simulink model "OfflineTestbench_OpenLoop"  (R2019b)
settings: Solver=ode1  StartTime=0.0  StopTime=30  FixedStep=0.01  RelTol=1e-3
PostLoadFcn:
  | , if any(exist('dsrtsu_mdlpostloadfcn', 'file') == [2, 3, 6]), try dsrtsu_mdlpostloadfcn('Execute', bdroot); catch fprintf('Error in PostLoadFcn (dsrtsu_mdlpostloadfcn) for model "%s":\n %s\n', bdroot, lasterr); end, end,
undefined symbols (not defined in the file): default_localization_bus, default_vehicle_state_bus, localization_testbed_matrix, MeasurementTime, Motion, Pose, Steering, time_testbed_vector, trajectory_testbed_matrix, vehicle_can_testbed_matrix
libraries: Lib_VehicleModel x3, Lib_Controller x1
settings Model: DSRTSU_INTERNAL_RTI_VER=550  DSRTSU_INTERNAL_RTI_TYPE=rti1401  RTICANMMDATA=struct('GeneralSetupData',struct('modelroot','C:\Users\kessler\Documents\fav\apollo_opensource\modules\autobox_control\models','generalsettings',struct('filesettings',struct('destfolder',struct('Name','RTICANMM_FILES','Check',1),'buildfolder',struct('Name','.','Check',1),'AbsDestfolder',struct('Name','C:\Users\kessler\Documents\fav\apollo_opensource\modules\autobox_control\models\RTICANMM_FILES'),'AbsBuildfolder',struct('Name','C:\Users\kessler\Documents\fav\apollo_opensource\modules\autobox_control\models'))),'options',struct('addpaths',1,'rmpaths',1,'addtrcexclusion',true,'cannavigator',struct('checkmonitoring',0),'show_usrtrc',0,'use_usrtrc',0),'advanced',struct('options',ones(1,100)),'MPSetup',{{}},'RTI',struct('Type','GRT','Ver','','Date',''),'modelname','OfflineTestbench_OpenLoop','block','OfflineTestbench_OpenLoop'))  DSRTSU_INTERNAL_RTIFPGA=150  Creator=esterle  LastModifiedBy=kessler
settings DataIOCC: ReturnWorkspaceOutputs=off
settings DebuggingCC: ArithmeticOperatorsInVariantConditions=warning
settings SFSimCC: SimUseLocalCustomCode=off  CustomCodeUndefinedFunction=UseInterfaceOnly
settings RTWCC: RTWUseLocalCustomCode=off

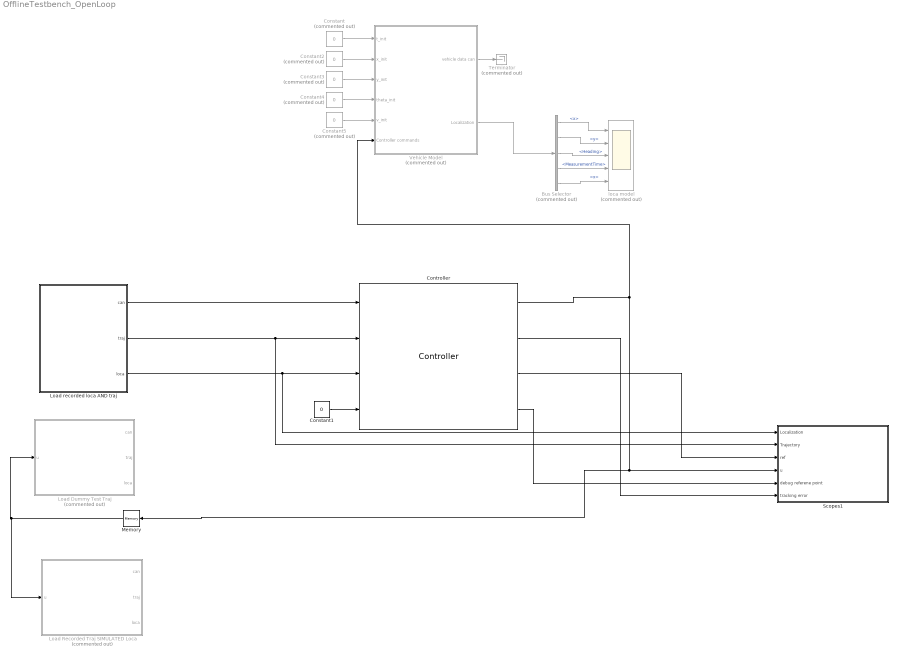
== system OfflineTestbench_OpenLoop ==
  Bus Selector : BusSelector  Commented=on  OutputSignals=Pose.Position.x,Pose.Position.y,Pose.Heading,MeasurementTime,Pose.LinearVelocity.x
  Constant{,2..5} (5 alike) : Constant  Commented=on  Value=0
  Constant1 : Constant  Value=0  OutDataTypeStr=boolean
  Controller : Lib_Controller/Controller  SystemSampleTime=-1  Latency=0  AutoFrameSizeCalculation=off
  Load Dummy Test Traj : Subsystem  Commented=on
  Load Recorded Traj SIMULATED Loca : Subsystem  Commented=on
  Load recorded loca AND traj : Subsystem
  Memory : Memory
  Scopes1 : Subsystem
  Terminator : Terminator  Commented=on
  Vehicle Model : Subsystem  Commented=on
  loca model : Scope  Commented=on  NumInputPorts=5
  wires:
  Constant1/1 -> Controller/4
  Controller/2 -> Scopes1/6(tracking error)
  Controller/1 -> Memory/1, Scopes1/4(u), Vehicle Model/6(Controller commands)
  Memory/1 -> Load Recorded Traj SIMULATED Loca/1(u), Load Dummy Test Traj/1(u)
  Controller/4 -> Scopes1/5(debug referene point)
  Controller/3 -> Scopes1/3(ref)
  Constant/1 -> Vehicle Model/1(t_init)
  Constant2/1 -> Vehicle Model/2(x_init)
  Constant3/1 -> Vehicle Model/3(y_init)
  Constant4/1 -> Vehicle Model/4(theta_init)
  Constant5/1 -> Vehicle Model/5(v_init)
  Vehicle Model/2(Localization) -> Bus Selector/1
  Vehicle Model/1(vehicle data can) -> Terminator/1
  Bus Selector/4 -> loca model/4  "<MeasurementTime>"
  Bus Selector/3 -> loca model/3  "<Heading>"
  Bus Selector/5 -> loca model/5  "<x>"
  Bus Selector/2 -> loca model/2  "<y>"
  Bus Selector/1 -> loca model/1  "<x>"
  Load recorded loca AND traj/2(traj) -> Scopes1/2(Trajectory), Controller/2
  Load recorded loca AND traj/3(loca) -> Scopes1/1(Localization), Controller/3
  Load recorded loca AND traj/1(can) -> Controller/1

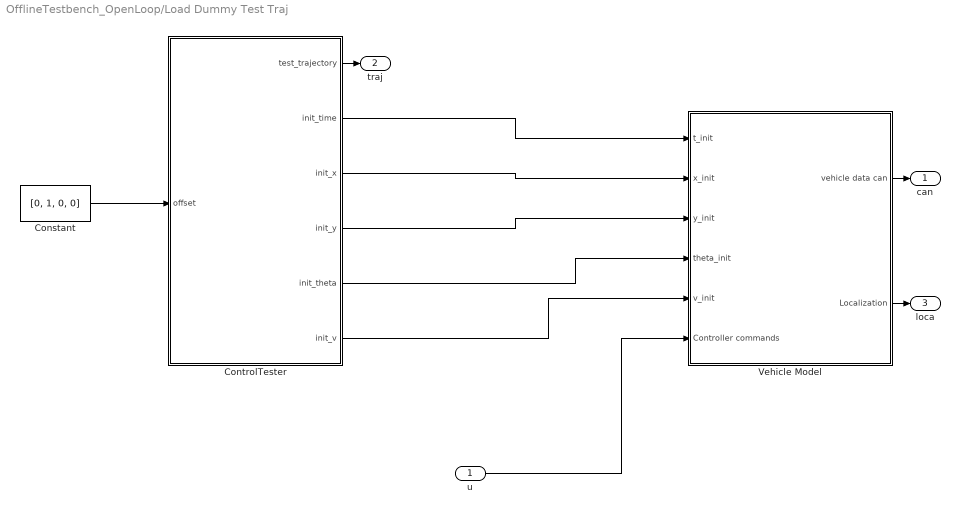
== system OfflineTestbench_OpenLoop/Load Dummy Test Traj ==
  u : Inport
  Constant : Constant  Value=[0, 1, 0, 0]
  "ControlTester " : MATLAB Function  TreatAsAtomicUnit=on
  Vehicle Model : Subsystem
  can : Outport  VectorParamsAs1DForOutWhenUnconnected=off
  traj : Outport  Port=2  VectorParamsAs1DForOutWhenUnconnected=off
  loca : Outport  Port=3  VectorParamsAs1DForOutWhenUnconnected=off
  wires:
  "ControlTester "/2(init_time) -> Vehicle Model/1(t_init)
  "ControlTester "/5(init_theta) -> Vehicle Model/4(theta_init)
  Constant/1 -> "ControlTester "/1(offset)
  "ControlTester "/6(init_v) -> Vehicle Model/5(v_init)
  "ControlTester "/3(init_x) -> Vehicle Model/2(x_init)
  "ControlTester "/4(init_y) -> Vehicle Model/3(y_init)
  "ControlTester "/1(test_trajectory) -> traj/1
  Vehicle Model/1(vehicle data can) -> can/1
  Vehicle Model/2(Localization) -> loca/1
  u/1 -> Vehicle Model/6(Controller commands)

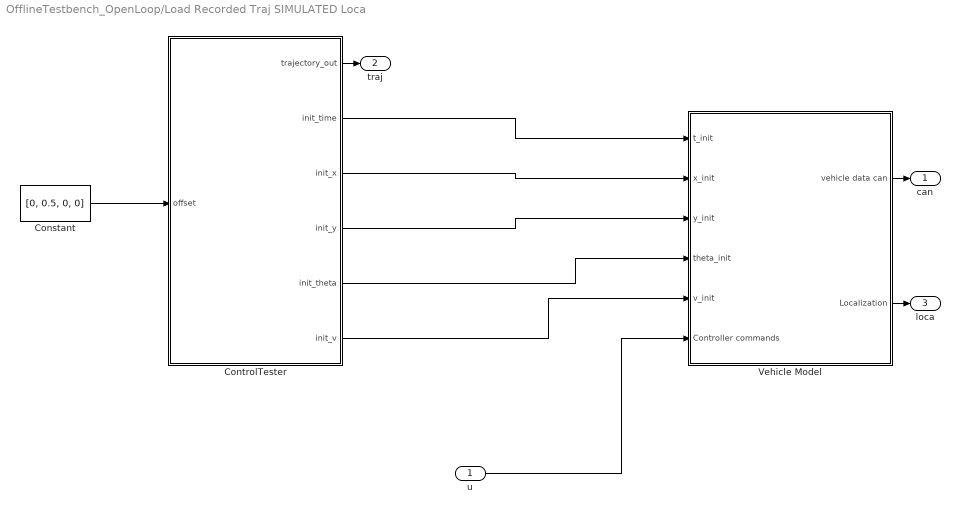
== system OfflineTestbench_OpenLoop/Load Recorded Traj SIMULATED Loca ==
  u : Inport
  Constant : Constant  Value=[0, 0.5, 0, 0]
  "ControlTester " : MATLAB Function  TreatAsAtomicUnit=on
  Vehicle Model : Subsystem
  can : Outport  VectorParamsAs1DForOutWhenUnconnected=off
  traj : Outport  Port=2  VectorParamsAs1DForOutWhenUnconnected=off
  loca : Outport  Port=3  VectorParamsAs1DForOutWhenUnconnected=off
  wires:
  u/1 -> Vehicle Model/6(Controller commands)
  Vehicle Model/2(Localization) -> loca/1
  Vehicle Model/1(vehicle data can) -> can/1
  "ControlTester "/1(trajectory_out) -> traj/1
  "ControlTester "/4(init_y) -> Vehicle Model/3(y_init)
  "ControlTester "/3(init_x) -> Vehicle Model/2(x_init)
  "ControlTester "/6(init_v) -> Vehicle Model/5(v_init)
  Constant/1 -> "ControlTester "/1(offset)
  "ControlTester "/5(init_theta) -> Vehicle Model/4(theta_init)
  "ControlTester "/2(init_time) -> Vehicle Model/1(t_init)

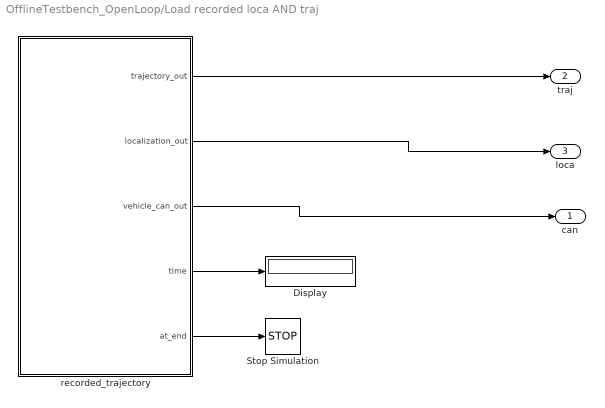
== system OfflineTestbench_OpenLoop/Load recorded loca AND traj ==
  Display : Display
  Stop Simulation : Stop
  recorded_trajectory : MATLAB Function  TreatAsAtomicUnit=on
  can : Outport  VectorParamsAs1DForOutWhenUnconnected=off
  traj : Outport  Port=2  VectorParamsAs1DForOutWhenUnconnected=off
  loca : Outport  Port=3  VectorParamsAs1DForOutWhenUnconnected=off
  wires:
  recorded_trajectory/5(at_end) -> Stop Simulation/1
  recorded_trajectory/4(time) -> Display/1
  recorded_trajectory/3(vehicle_can_out) -> can/1
  recorded_trajectory/2(localization_out) -> loca/1
  recorded_trajectory/1(trajectory_out) -> traj/1

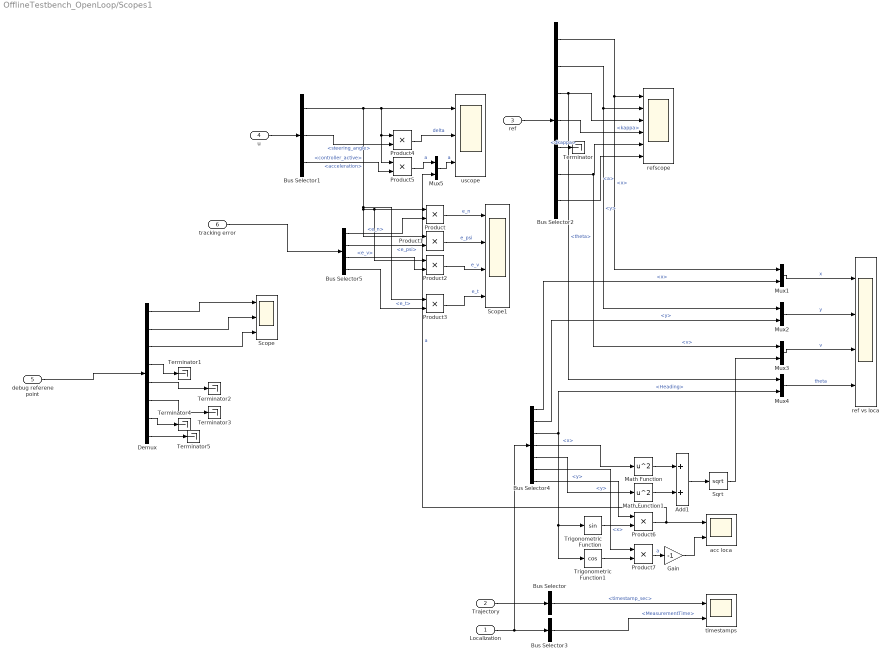
== system OfflineTestbench_OpenLoop/Scopes1 ==
  Localization : Inport  OutDataTypeStr=Bus: LocalizationToAutobox  BusOutputAsStruct=on
  Trajectory : Inport  Port=2  OutDataTypeStr=Bus: ControlTrajectory  BusOutputAsStruct=on
  ref : Inport  Port=3
  u : Inport  Port=4
  debug referene point : Inport  Port=5
  tracking error : Inport  Port=6
  Add1 : Sum
  Bus Selector : BusSelector  OutputSignals=timestamp_sec
  Bus Selector1 : BusSelector  OutputSignals=controller_active,steering_angle,acceleration
  Bus Selector2 : BusSelector  OutputSignals=x,y,theta,kappa,dkappa,v,a
  Bus Selector3 : BusSelector  OutputSignals=MeasurementTime
  Bus Selector4 : BusSelector  OutputSignals=Pose.Position.x,Pose.Position.y,Pose.Heading,Pose.LinearVelocity.x,Pose.LinearVelocity.y,Pose.LinearAcceleration.x,Pose.LinearAcceleration.y
  Bus Selector5 : BusSelector  OutputSignals=e_n,e_psi,e_v,e_t
  Demux : Demux  Outputs=8
  Gain : Gain  Gain=-1
  Math Function : Math  Operator=square  SaturateOnIntegerOverflow=on
  Math Function1 : Math  Operator=square  SaturateOnIntegerOverflow=on
  Mux{1..5} (5 alike) : Mux  Inputs=2
  Product{,1..7} (8 alike) : Product
  Scope : Scope  NumInputPorts=3
  Scope1 : Scope  NumInputPorts=4
  Sqrt : Sqrt  SaturateOnIntegerOverflow=on
  Terminator{,1..5} (6 alike) : Terminator
  Trigonometric Function : Trigonometry
  Trigonometric Function1 : Trigonometry  Operator=cos
  acc loca : Scope  NumInputPorts=2
  ref vs loca : Scope  NumInputPorts=4
  refscope : Scope  NumInputPorts=6
  timestamps : Scope  NumInputPorts=2
  uscope : Scope  NumInputPorts=3
  wires:
  Bus Selector1/1 -> Product3/1, Product2/1, Product/1, Product1/1, Product5/1, Product4/1, uscope/1  "<controller_active>"
  Bus Selector1/2 -> Product4/2  "<steering_angle>"
  Bus Selector1/3 -> Product5/2  "<acceleration>"
  Bus Selector2/5 -> Terminator/1  "<dkappa>"
  u/1 -> Bus Selector1/1
  ref/1 -> Bus Selector2/1
  Bus Selector2/4 -> refscope/4  "<kappa>"
  Bus Selector2/3 -> Mux4/1, refscope/3  "<theta>"
  Bus Selector2/1 -> Mux1/1, refscope/1  "<x>"
  Bus Selector2/6 -> Mux3/1, refscope/5  "<v>"
  Bus Selector2/7 -> refscope/6  "<a>"
  Bus Selector2/2 -> Mux2/1, refscope/2  "<y>"
  Trajectory/1 -> Bus Selector/1
  Localization/1 -> Bus Selector4/1, Bus Selector3/1
  Bus Selector3/1 -> timestamps/2  "<MeasurementTime>"
  Bus Selector/1 -> timestamps/1  "<timestamp_sec>"
  Mux4/1 -> ref vs loca/4  "theta"
  Mux2/1 -> ref vs loca/2  "y"
  Mux3/1 -> ref vs loca/3  "v"
  Mux1/1 -> ref vs loca/1  "x"
  Bus Selector4/1 -> Mux1/2  "<x>"
  Bus Selector4/2 -> Mux2/2  "<y>"
  Bus Selector4/3 -> Mux4/2, Trigonometric Function1/1, Trigonometric Function/1  "<Heading>"
  Math Function1/1 -> Add1/2
  Math Function/1 -> Add1/1
  Add1/1 -> Sqrt/1
  Bus Selector4/4 -> Math Function/1  "<x>"
  Bus Selector4/5 -> Math Function1/1  "<y>"
  Sqrt/1 -> Mux3/2
  Demux/3 -> Scope/3
  Demux/1 -> Scope/1
  Demux/2 -> Scope/2
  debug referene point/1 -> Demux/1
  Bus Selector5/2 -> Product1/2  "<e_psi>"
  Bus Selector5/4 -> Product3/2  "<e_t>"
  Bus Selector5/3 -> Product2/2  "<e_v>"
  Bus Selector5/1 -> Product/2  "<e_n>"
  tracking error/1 -> Bus Selector5/1
  Demux/4 -> Terminator1/1
  Demux/5 -> Terminator2/1
  Demux/6 -> Terminator3/1
  Demux/7 -> Terminator4/1
  Demux/8 -> Terminator5/1
  Product/1 -> Scope1/1  "e_n"
  Product1/1 -> Scope1/2  "e_psi"
  Product2/1 -> Scope1/3  "e_v"
  Product3/1 -> Scope1/4  "e_t"
  Product4/1 -> uscope/2  "delta"
  Product5/1 -> Mux5/1  "a"
  Mux5/1 -> uscope/3  "a"
  Trigonometric Function/1 -> Product6/2
  Bus Selector4/7 -> Product6/1  "<y>"
  Bus Selector4/6 -> Product7/1  "<x>"
  Trigonometric Function1/1 -> Product7/2
  Product6/1 -> Mux5/2, acc loca/1  "a"
  Product7/1 -> Gain/1  "a"
  Gain/1 -> acc loca/2

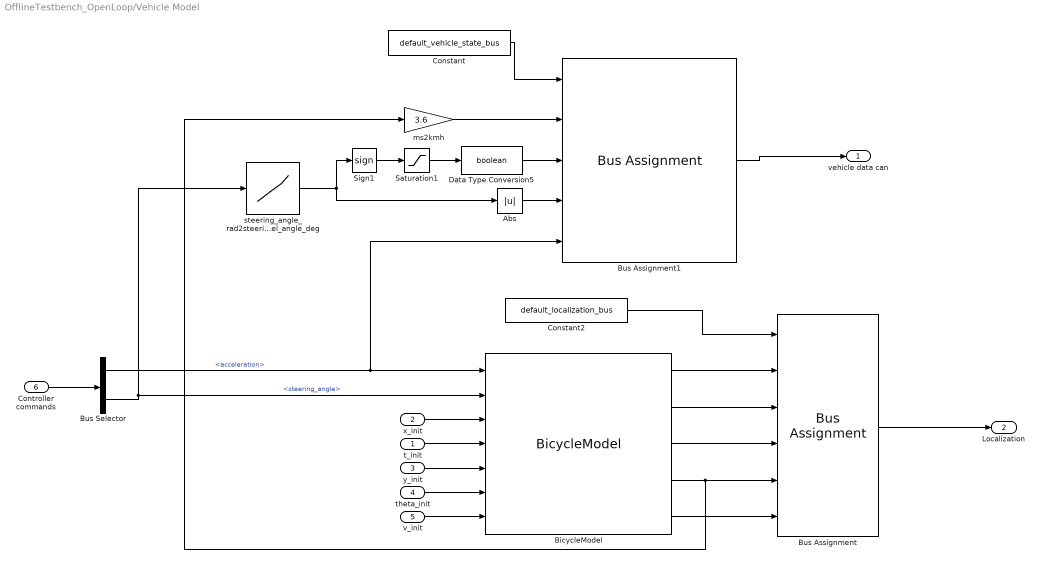
== system OfflineTestbench_OpenLoop/Vehicle Model ==
  t_init : Inport
  x_init : Inport  Port=2
  y_init : Inport  Port=3
  theta_init : Inport  Port=4
  v_init : Inport  Port=5
  Controller commands : Inport  Port=6
  Abs : Abs
  BicycleModel : Lib_VehicleModel/BicycleModel  l=2.6
  Bus Assignment : BusAssignment  AssignedSignals=Pose.Position.x,Pose.Position.y,Pose.Heading,Pose.LinearVelocity.x,MeasurementTime
  Bus Assignment1 : BusAssignment  AssignedSignals=Motion.VehicleVelocity,Steering.SteeringWheelAngleSign,Steering.SteeringWheelAngle,Motion.LongitudinalAcceleration
  Bus Selector : BusSelector  OutputSignals=acceleration,steering_angle
  Constant : Constant  Value=default_vehicle_state_bus  OutDataTypeStr=Bus: vehicle_data_can_bus
  Constant2 : Constant  Value=default_localization_bus  OutDataTypeStr=Bus: LocalizationToAutobox
  Data Type Conversion5 : DataTypeConversion  OutDataTypeStr=boolean
  Saturation1 : Saturate  UpperLimit=1  LowerLimit=0
  Sign1 : Signum
  ms2kmh : Gain  Gain=3.6
  steering_angle_rad2steering_wheel_angle_deg : Lookup_n-D  NumberOfTableDimensions=1  BreakpointsForDimension1=[-0.62 0 0.62]  Table=[-400, 0, 400]  InternalRulePriority=Speed  RndMeth=Simplest  InputSameDT=on
  vehicle data can : Outport  VectorParamsAs1DForOutWhenUnconnected=off
  Localization : Outport  Port=2  VectorParamsAs1DForOutWhenUnconnected=off
  wires:
  Controller commands/1 -> Bus Selector/1
  Bus Assignment/1 -> Localization/1
  Bus Selector/1 -> Bus Assignment1/5, BicycleModel/1  "<acceleration>"
  Bus Selector/2 -> BicycleModel/2, steering_angle_rad2steering_wheel_angle_deg/1  "<steering_angle>"
  BicycleModel/5 -> Bus Assignment/6
  y_init/1 -> BicycleModel/5
  BicycleModel/2 -> Bus Assignment/3
  BicycleModel/1 -> Bus Assignment/2
  BicycleModel/3 -> Bus Assignment/4
  v_init/1 -> BicycleModel/7
  theta_init/1 -> BicycleModel/6
  x_init/1 -> BicycleModel/3
  Constant2/1 -> Bus Assignment/1
  BicycleModel/4 -> Bus Assignment/5, ms2kmh/1
  t_init/1 -> BicycleModel/4
  Data Type Conversion5/1 -> Bus Assignment1/3
  Abs/1 -> Bus Assignment1/4
  Saturation1/1 -> Data Type Conversion5/1
  Sign1/1 -> Saturation1/1
  ms2kmh/1 -> Bus Assignment1/2
  steering_angle_rad2steering_wheel_angle_deg/1 -> Abs/1, Sign1/1
  Constant/1 -> Bus Assignment1/1
  Bus Assignment1/1 -> vehicle data can/1

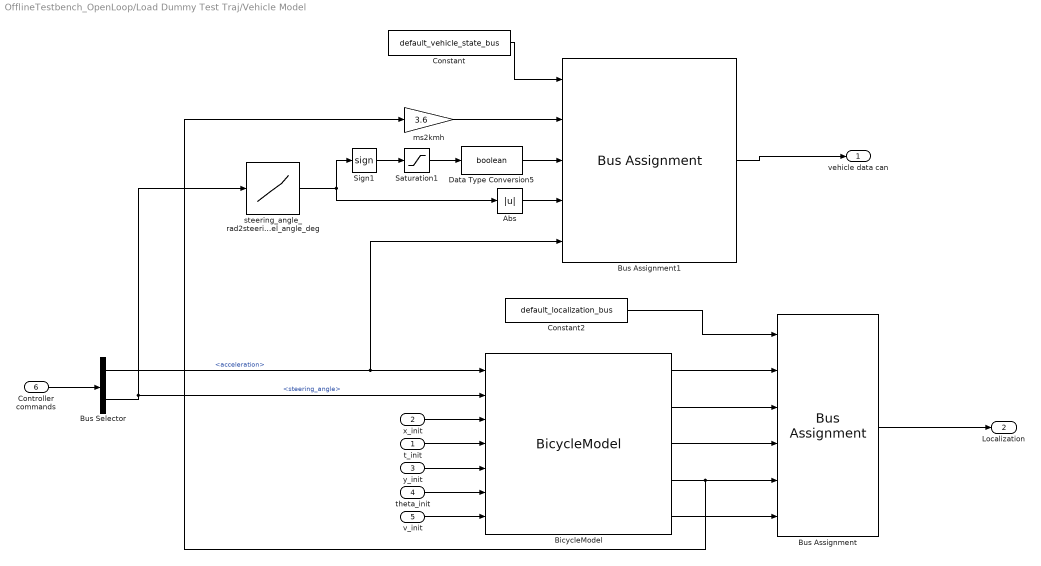
== system OfflineTestbench_OpenLoop/Load Dummy Test Traj/Vehicle Model ==
  t_init : Inport
  x_init : Inport  Port=2
  y_init : Inport  Port=3
  theta_init : Inport  Port=4
  v_init : Inport  Port=5
  Controller commands : Inport  Port=6
  Abs : Abs
  BicycleModel : Lib_VehicleModel/BicycleModel  l=2.6
  Bus Assignment : BusAssignment  AssignedSignals=Pose.Position.x,Pose.Position.y,Pose.Heading,Pose.LinearVelocity.x,MeasurementTime
  Bus Assignment1 : BusAssignment  AssignedSignals=Motion.VehicleVelocity,Steering.SteeringWheelAngleSign,Steering.SteeringWheelAngle,Motion.LongitudinalAcceleration
  Bus Selector : BusSelector  OutputSignals=acceleration,steering_angle
  Constant : Constant  Value=default_vehicle_state_bus  OutDataTypeStr=Bus: vehicle_data_can_bus
  Constant2 : Constant  Value=default_localization_bus  OutDataTypeStr=Bus: LocalizationToAutobox
  Data Type Conversion5 : DataTypeConversion  OutDataTypeStr=boolean
  Saturation1 : Saturate  UpperLimit=1  LowerLimit=0
  Sign1 : Signum
  ms2kmh : Gain  Gain=3.6
  steering_angle_rad2steering_wheel_angle_deg : Lookup_n-D  NumberOfTableDimensions=1  BreakpointsForDimension1=[-0.62 0 0.62]  Table=[-400, 0, 400]  InternalRulePriority=Speed  RndMeth=Simplest  InputSameDT=on
  vehicle data can : Outport  VectorParamsAs1DForOutWhenUnconnected=off
  Localization : Outport  Port=2  VectorParamsAs1DForOutWhenUnconnected=off
  wires:
  Controller commands/1 -> Bus Selector/1
  Bus Assignment/1 -> Localization/1
  Bus Selector/1 -> Bus Assignment1/5, BicycleModel/1  "<acceleration>"
  Bus Selector/2 -> BicycleModel/2, steering_angle_rad2steering_wheel_angle_deg/1  "<steering_angle>"
  BicycleModel/5 -> Bus Assignment/6
  y_init/1 -> BicycleModel/5
  BicycleModel/2 -> Bus Assignment/3
  BicycleModel/1 -> Bus Assignment/2
  BicycleModel/3 -> Bus Assignment/4
  v_init/1 -> BicycleModel/7
  theta_init/1 -> BicycleModel/6
  x_init/1 -> BicycleModel/3
  Constant2/1 -> Bus Assignment/1
  BicycleModel/4 -> Bus Assignment/5, ms2kmh/1
  t_init/1 -> BicycleModel/4
  Data Type Conversion5/1 -> Bus Assignment1/3
  Abs/1 -> Bus Assignment1/4
  Saturation1/1 -> Data Type Conversion5/1
  Sign1/1 -> Saturation1/1
  ms2kmh/1 -> Bus Assignment1/2
  steering_angle_rad2steering_wheel_angle_deg/1 -> Abs/1, Sign1/1
  Constant/1 -> Bus Assignment1/1
  Bus Assignment1/1 -> vehicle data can/1

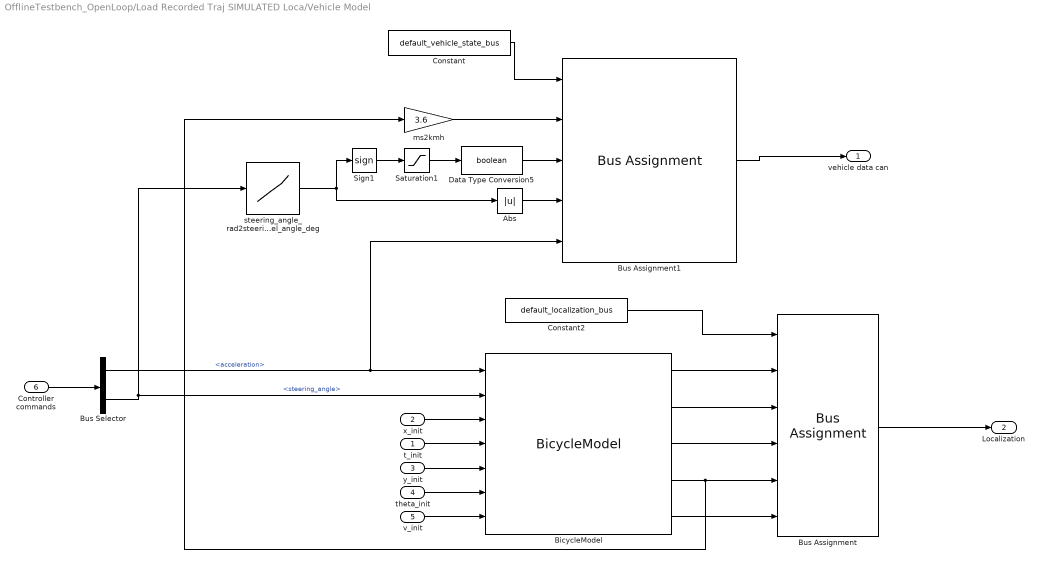
== system OfflineTestbench_OpenLoop/Load Recorded Traj SIMULATED Loca/Vehicle Model ==
  t_init : Inport
  x_init : Inport  Port=2
  y_init : Inport  Port=3
  theta_init : Inport  Port=4
  v_init : Inport  Port=5
  Controller commands : Inport  Port=6
  Abs : Abs
  BicycleModel : Lib_VehicleModel/BicycleModel  l=2.6
  Bus Assignment : BusAssignment  AssignedSignals=Pose.Position.x,Pose.Position.y,Pose.Heading,Pose.LinearVelocity.x,MeasurementTime
  Bus Assignment1 : BusAssignment  AssignedSignals=Motion.VehicleVelocity,Steering.SteeringWheelAngleSign,Steering.SteeringWheelAngle,Motion.LongitudinalAcceleration
  Bus Selector : BusSelector  OutputSignals=acceleration,steering_angle
  Constant : Constant  Value=default_vehicle_state_bus  OutDataTypeStr=Bus: vehicle_data_can_bus
  Constant2 : Constant  Value=default_localization_bus  OutDataTypeStr=Bus: LocalizationToAutobox
  Data Type Conversion5 : DataTypeConversion  OutDataTypeStr=boolean
  Saturation1 : Saturate  UpperLimit=1  LowerLimit=0
  Sign1 : Signum
  ms2kmh : Gain  Gain=3.6
  steering_angle_rad2steering_wheel_angle_deg : Lookup_n-D  NumberOfTableDimensions=1  BreakpointsForDimension1=[-0.62 0 0.62]  Table=[-400, 0, 400]  InternalRulePriority=Speed  RndMeth=Simplest  InputSameDT=on
  vehicle data can : Outport  VectorParamsAs1DForOutWhenUnconnected=off
  Localization : Outport  Port=2  VectorParamsAs1DForOutWhenUnconnected=off
  wires:
  Bus Assignment1/1 -> vehicle data can/1
  Constant/1 -> Bus Assignment1/1
  steering_angle_rad2steering_wheel_angle_deg/1 -> Sign1/1, Abs/1
  ms2kmh/1 -> Bus Assignment1/2
  Sign1/1 -> Saturation1/1
  Saturation1/1 -> Data Type Conversion5/1
  Abs/1 -> Bus Assignment1/4
  Data Type Conversion5/1 -> Bus Assignment1/3
  t_init/1 -> BicycleModel/4
  BicycleModel/4 -> ms2kmh/1, Bus Assignment/5
  Constant2/1 -> Bus Assignment/1
  x_init/1 -> BicycleModel/3
  theta_init/1 -> BicycleModel/6
  v_init/1 -> BicycleModel/7
  BicycleModel/3 -> Bus Assignment/4
  BicycleModel/1 -> Bus Assignment/2
  BicycleModel/2 -> Bus Assignment/3
  y_init/1 -> BicycleModel/5
  BicycleModel/5 -> Bus Assignment/6
  Bus Selector/2 -> steering_angle_rad2steering_wheel_angle_deg/1, BicycleModel/2  "<steering_angle>"
  Bus Selector/1 -> BicycleModel/1, Bus Assignment1/5  "<acceleration>"
  Bus Assignment/1 -> Localization/1
  Controller commands/1 -> Bus Selector/1

== matlab function OfflineTestbench_OpenLoop/Load Dummy Test Traj/ControlTester  ==
  data: test_trajectory output Bus: ControlTrajectory; init_time output; init_x output; init_y output; init_theta output; init_v output; offset input
function [test_trajectory, init_time, init_x, init_y, init_theta, init_v]  = ControlTester(offset)
coder.extrinsic('display')
persistent test_number;

test_trajectory = struct('n_trajectory_point',uint32(0),'x',zeros(1000,1), 'y',zeros(1000,1), ...
    'z', zeros(1000,1), 'theta', zeros(1000,1),'kappa',zeros(1000,1),...
    'dkappa', zeros(1000,1),'ddkappa', zeros(1000,1),'s',zeros(1000,1),...
    'v',zeros(1000,1),'a', zeros(1000,1),'relative_time',zeros(1000,1),...
    'timestamp_sec', zeros(1,1));

point3d = struct('x',double(0),'y',double(0),'z',double(0));
point_enu= struct('x',double(0),'y',double(0),'z',double(0));
quaternion = struct('qx',double(0),'qy',double(0),'qz',double(0),'qw',double(0));
pose = struct('Position',point_enu,'Orientation',quaternion,...
    'LinearVelocity',point3d,'LinearAcceleration',point3d, 'AngularVelocity',point3d,'Heading',double(0),...
    'LinearAccelerationVrf',point3d,'AngularVelocityVrf',point3d,'EulerAngles',point3d);
uncertainty = struct('PositionStdDev',point3d,'OrientationStdDev',point3d,...
'LinearVelocityStdDev',point3d,'LinearAccelerationStdDev',point3d,'AngularVelocityStdDev',point3d);

if isempty(test_number)
    test_number=0;
end



temp = load('trajectory.mat');
pb_trajectory = temp.trajectory;


test_trajectory.n_trajectory_point = uint32(size(pb_trajectory.x,2));    
test_trajectory.x = pb_trajectory.x';
test_trajectory.y = pb_trajectory.y';
test_trajectory.z = pb_trajectory.z';
test_trajectory.theta = pb_trajectory.theta';
test_trajectory.kappa = pb_trajectory.curvature';
test_trajectory.dkappa = pb_trajectory.curvature_change_rate';
%trajectory.ddkappa = zeros(1000,1); todo remove from bus -> not used
%by controller
test_trajectory.v = pb_trajectory.speed';
test_trajectory.a = pb_trajectory.acceleration_s';
test_trajectory.relative_time = pb_trajectory.relative_time';
test_trajectory.timestamp_sec = pb_trajectory.header.timestamp_sec;

init_time = test_trajectory.timestamp_sec;
init_x = test_trajectory.x(1)+offset(1);
init_y = test_trajectory.y(1)+offset(2);
init_theta = test_trajectory.theta(1)+offset(3);
init_v = test_trajectory.v(1)+offset(4);

== matlab function OfflineTestbench_OpenLoop/Load recorded loca AND traj/recorded_trajectory ==
  data: trajectory_out output Bus: ControlTrajectory; localization_out output Bus: LocalizationToAutobox; vehicle_can_out output Bus: vehicle_data_can_bus; time output; at_end output; time_testbed_vector parameter; trajectory_testbed_matrix parameter; localization_testbed_matrix parameter; vehicle_can_testbed_matrix parameter
function [trajectory_out, localization_out, vehicle_can_out, time, at_end]   = recorded_trajectory(  time_testbed_vector, trajectory_testbed_matrix, localization_testbed_matrix, vehicle_can_testbed_matrix)
coder.extrinsic('num2str');
coder.extrinsic('getfield');
coder.extrinsic('load');
coder.extrinsic('evalin');
coder.extrinsic('assignin');
coder.extrinsic('default_vehicle_state_bus');
coder.extrinsic('boolean');

persistent current_idx;
if isempty(current_idx)
    current_idx = 0;
end
current_idx = current_idx + 1;

point3d = struct('x',double(0),'y',double(0),'z',double(0));
point_enu= struct('x',double(0),'y',double(0),'z',double(0));
quaternion = struct('qx',double(0),'qy',double(0),'qz',double(0),'qw',double(0));
pose = struct('Position',point_enu,'Orientation',quaternion,...
    'LinearVelocity',point3d,'LinearAcceleration',point3d, 'AngularVelocity',point3d,'Heading',double(0),...
    'LinearAccelerationVrf',point3d,'AngularVelocityVrf',point3d,'EulerAngles',point3d);
uncertainty = struct('PositionStdDev',point3d,'OrientationStdDev',point3d,...
'LinearVelocityStdDev',point3d,'LinearAccelerationStdDev',point3d,'AngularVelocityStdDev',point3d);

localization_out = struct('Pose', pose, 'MeasurementTime', double(0), 'Uncertainty', uncertainty);
trajectory_out = struct('n_trajectory_point',uint32(0),'x',zeros(1000,1), 'y',zeros(1000,1), ...
    'z', zeros(1000,1), 'theta', zeros(1000,1),'kappa',zeros(1000,1),...
    'dkappa', zeros(1000,1),'ddkappa', zeros(1000,1),'s',zeros(1000,1),...
    'v',zeros(1000,1),'a', zeros(1000,1),'relative_time',zeros(1000,1),...
    'timestamp_sec', zeros(1,1));

vehicle_can_out = evalin('base','default_vehicle_state_bus');

at_end = false;
time = double(0);

%endidx = double(0);
endidx = length(time_testbed_vector);
if(current_idx >= endidx)
    at_end = true;
else

time = time_testbed_vector(current_idx);

tv = trajectory_testbed_matrix(:,current_idx);
lv = localization_testbed_matrix(:,current_idx);
cv = vehicle_can_testbed_matrix(:,current_idx);


trajectory_out.n_trajectory_point = uint32(tv(1));
trajectory_out.timestamp_sec = tv(2);
trajectory_out.a = tv(3:1002);
trajectory_out.ddkappa = tv(1003:2002);
trajectory_out.dkappa = tv(2003:3002); 
trajectory_out.kappa = tv(3003:4002);
trajectory_out.relative_time = tv(4003:5002);
trajectory_out.s  = tv(5003:6002);
trajectory_out.theta = tv(6003:7002);
trajectory_out.v = tv(7003:8002);
trajectory_out.x = tv(8003:9002);
trajectory_out.y = tv(9003:10002);
trajectory_out.z = tv(10003:11002);

localization_out.MeasurementTime = lv(1);
localization_out.Pose.AngularVelocity.x = lv(2);
localization_out.Pose.AngularVelocity.y = lv(3);
localization_out.Pose.AngularVelocity.z = lv(4);
localization_out.Pose.AngularVelocityVrf.x = lv(5);
localization_out.Pose.AngularVelocityVrf.y = lv(6);
localization_out.Pose.AngularVelocityVrf.z = lv(7);
localization_out.Pose.EulerAngles.x = lv(8);
localization_out.Pose.EulerAngles.y = lv(9);
localization_out.Pose.EulerAngles.z = lv(10);
localization_out.Pose.Heading = lv(11);
localization_out.Pose.LinearAcceleration.x = lv(12);
localization_out.Pose.LinearAcceleration.y = lv(13);
localization_out.Pose.LinearAcceleration.z = lv(14);
localization_out.Pose.LinearAccelerationVrf.x = lv(15);
localization_out.Pose.LinearAccelerationVrf.y = lv(16);
localization_out.Pose.LinearAccelerationVrf.z = lv(17);
localization_out.Pose.LinearVelocity.x = lv(18);
localization_out.Pose.LinearVelocity.y = lv(19);
localization_out.Pose.LinearVelocity.z = lv(20);
localization_out.Pose.Orientation.qw = lv(21);
localization_out.Pose.Orientation.qx = lv(22);
localization_out.Pose.Orientation.qy = lv(23);
localization_out.Pose.Orientation.qz = lv(24);
localization_out.Pose.Position.x = lv(25);
localization_out.Pose.Position.y = lv(26);
localization_out.Pose.Position.z = lv(27);

vehicle_can_out.Motion.CRC = uint8(cv(1));
vehicle_can_out.Motion.Counter = uint8(cv(2));
vehicle_can_out.Motion.LateralAcceleration = cv(3);
vehicle_can_out.Motion.LongitudinalAcceleration = cv(4);
vehicle_can_out.Motion.VehicleVelocity = cv(5);
vehicle_can_out.Motion.YawRate = cv(6);
vehicle_can_out.Motion.YawRateSign = boolean(cv(7));
vehicle_can_out.Steering.CRC = uint8(cv(8));
vehicle_can_out.Steering.Counter = uint8(cv(9));
vehicle_can_out.Steering.SteeringWheelAngle = cv(10);
vehicle_can_out.Steering.SteeringWheelAngleSign = boolean(cv(11));
vehicle_can_out.Steering.SteeringWheelSpeed = uint16(cv(12));
vehicle_can_out.Steering.SteeringWheelSpeedSign = boolean(cv(13));
vehicle_can_out.Steering.SteeringWheelTorque = cv(14);
vehicle_can_out.Steering.SteeringWheelTorqueSign = boolean(cv(15));

end


%assignin('base','idxtmp',1)
%[trajectory, localization, vehicle_data_can] = evalin('base','getRecordedStateAtIndex(cda, idxtmp)');
%trajectory_out = trajectory;
%localization_out.Pose = localization.Pose;
%localization_out.MeasurementTime = localization.MeasurementTime;
%vehicle_can_out = vehicle_data_can;



%assignin('base','time',time)
%trajectory_out = evalin('base', 'lt.trajectory_bus(time)');
%localization_out.MeasurementTime = evalin('base', 'lt.localization_bus(time).MeasurementTime');
%localization_out.Pose.Position.x = evalin('base', 'lt.localization_bus(time).Pose.Position.x');
%localization_out.Pose.Position.y = evalin('base', 'lt.localization_bus(time).Pose.Position.y');
%localization_out.Pose.EulerAngles.z = evalin('base', 'lt.localization_bus(time).Pose.EulerAngles.z');

== matlab function OfflineTestbench_OpenLoop/Load Recorded Traj SIMULATED Loca/ControlTester  ==
  data: trajectory_out output Bus: ControlTrajectory; init_time output; init_x output; init_y output; init_theta output; init_v output; offset input; trajectory_testbed_matrix parameter
function [trajectory_out, init_time, init_x, init_y, init_theta, init_v]  = ControlTester(offset, trajectory_testbed_matrix)

trajectory_out = struct('n_trajectory_point',uint32(0),'x',zeros(1000,1), 'y',zeros(1000,1), ...
    'z', zeros(1000,1), 'theta', zeros(1000,1),'kappa',zeros(1000,1),...
    'dkappa', zeros(1000,1),'ddkappa', zeros(1000,1),'s',zeros(1000,1),...
    'v',zeros(1000,1),'a', zeros(1000,1),'relative_time',zeros(1000,1),...
    'timestamp_sec', zeros(1,1));

point3d = struct('x',double(0),'y',double(0),'z',double(0));
point_enu= struct('x',double(0),'y',double(0),'z',double(0));
quaternion = struct('qx',double(0),'qy',double(0),'qz',double(0),'qw',double(0));
pose = struct('Position',point_enu,'Orientation',quaternion,...
    'LinearVelocity',point3d,'LinearAcceleration',point3d, 'AngularVelocity',point3d,'Heading',double(0),...
    'LinearAccelerationVrf',point3d,'AngularVelocityVrf',point3d,'EulerAngles',point3d);
uncertainty = struct('PositionStdDev',point3d,'OrientationStdDev',point3d,...
'LinearVelocityStdDev',point3d,'LinearAccelerationStdDev',point3d,'AngularVelocityStdDev',point3d);


current_idx = 163;

tv = trajectory_testbed_matrix(:,current_idx);

trajectory_out.n_trajectory_point = uint32(tv(1));
trajectory_out.timestamp_sec = tv(2);
trajectory_out.a = tv(3:1002);
trajectory_out.ddkappa = tv(1003:2002);
trajectory_out.dkappa = tv(2003:3002); 
trajectory_out.kappa = tv(3003:4002);
trajectory_out.relative_time = tv(4003:5002);
trajectory_out.s  = tv(5003:6002);
trajectory_out.theta = tv(6003:7002);
trajectory_out.v = tv(7003:8002);
trajectory_out.x = tv(8003:9002);
trajectory_out.y = tv(9003:10002);
trajectory_out.z = tv(10003:11002);


init_time = trajectory_out.timestamp_sec;
init_x = trajectory_out.x(1)+offset(1);
init_y = trajectory_out.y(1)+offset(2);
init_theta = trajectory_out.theta(1)+offset(3);
init_v = trajectory_out.v(1)+offset(4);
